simulink model "stt_feedback_integral_action"  (R2022a)
settings: Solver=VariableStepAuto  StartTime=0.0  StopTime=Tsim  RelTol=1e-3
values from neighbouring files (symbols this model uses):
  H = Ka(size(A,1)+1:end)    [code6_continuous_augmented.m]
  K = Ka(1:size(A,1))    [code6_continuous_augmented.m]
undefined symbols (not defined in the file or in its folder): A, B, C, D
settings Model: Creator=aaron  LastModifiedBy=aaron

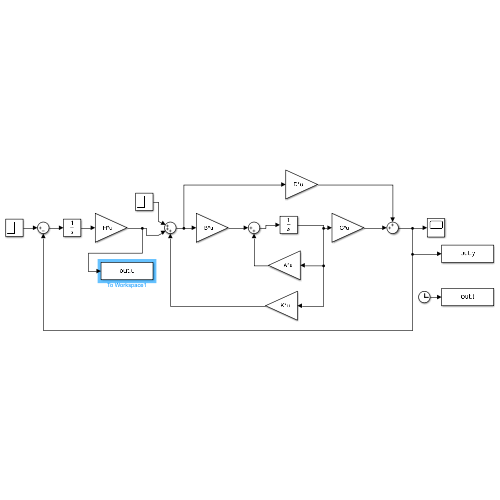
[thumbnail: Simulink's stored preview of the top-level diagram]
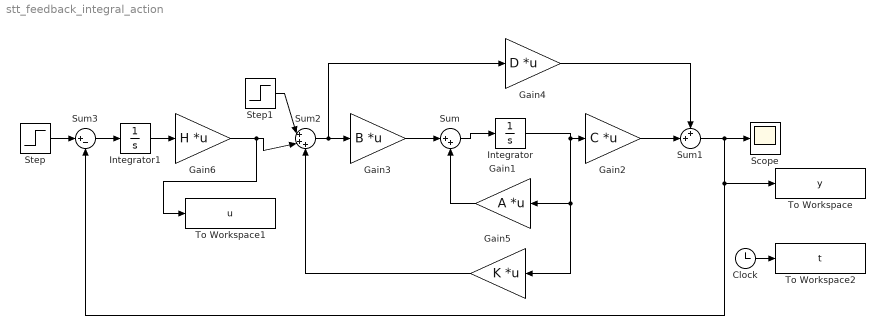
== system stt_feedback_integral_action ==
  Clock : Clock
  Gain1 : Gain  Gain=A  Multiplication=Matrix(K*u)
  Gain2 : Gain  Gain=C  Multiplication=Matrix(K*u)
  Gain3 : Gain  Gain=B  Multiplication=Matrix(K*u)
  Gain4 : Gain  Gain=D  Multiplication=Matrix(K*u)
  Gain5 : Gain  Gain=K  Multiplication=Matrix(K*u)
  Gain6 : Gain  Gain=H  Multiplication=Matrix(K*u)
  Integrator : Integrator
  Integrator1 : Integrator
  Scope : Scope
  Step : Step  SampleTime=0
  Step1 : Step  Time=15  SampleTime=0
  Sum : Sum  Inputs=|++
  Sum1 : Sum  Inputs=++|
  Sum2 : Sum  Inputs=|+++
  Sum3 : Sum  Inputs=|+-
  To Workspace : ToWorkspace  VariableName=y  SampleTime=-1
  To Workspace1 : ToWorkspace  VariableName=u  SampleTime=-1
  To Workspace2 : ToWorkspace  VariableName=t  SampleTime=-1
  wires:
  Integrator/1 -> Gain5/1, Gain1/1, Gain2/1
  Sum/1 -> Integrator/1
  Gain1/1 -> Sum/2
  Gain3/1 -> Sum/1
  Gain2/1 -> Sum1/2
  Gain4/1 -> Sum1/1
  Sum2/1 -> Gain4/1, Gain3/1
  Gain5/1 -> Sum2/3
  Gain6/1 -> To Workspace1/1, Sum2/2
  Integrator1/1 -> Gain6/1
  Sum3/1 -> Integrator1/1
  Sum1/1 -> Scope/1, To Workspace/1, Sum3/2
  Step/1 -> Sum3/1
  Step1/1 -> Sum2/1
  Clock/1 -> To Workspace2/1
